simulink model "msd_sl_ctl"  (R2021b)
settings: Solver=VariableStepAuto  StartTime=0.0  StopTime=20.0  RelTol=1e-3
values from neighbouring files (symbols this model uses):
  A = [0 1; -k/m -c/m]    [msd_sl_ctrl_design.m]
  B = [0; 1/m]    [msd_sl_ctrl_design.m]
  K1 = 5    [msd_sl_ctrl_design.m]
  S = smcplace(A,B,P)    [msd_sl_ctrl_design.m]    (also in smcplace.m = [place(A11,A12,P) eye(Bcol)])
settings Model: Creator=shohei  LastModifiedBy=shohei

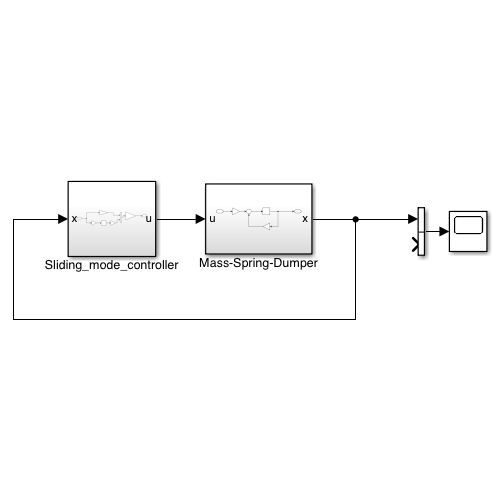
[thumbnail: Simulink's stored preview of the top-level diagram]
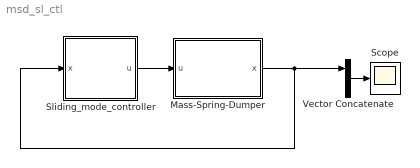
== system msd_sl_ctl ==
  Mass-Spring-Dumper : Subsystem
  Scope : Scope
  Sliding_mode_controller : Subsystem
  Vector Concatenate : Concatenate
  wires:
  Mass-Spring-Dumper/1(x) -> Sliding_mode_controller/1(x), Vector Concatenate/1
  Sliding_mode_controller/1(u) -> Mass-Spring-Dumper/1(u)
  Vector Concatenate/1 -> Scope/1

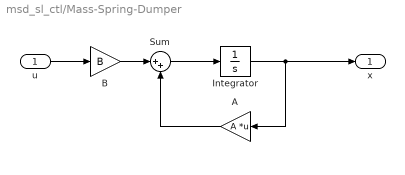
== system msd_sl_ctl/Mass-Spring-Dumper ==
  u : Inport
  A : Gain  Gain=A  Multiplication=Matrix(K*u)
  B : Gain  Gain=B
  Integrator : Integrator
  Sum : Sum  Inputs=|++
  x : Outport
  wires:
  u/1 -> B/1
  Sum/1 -> Integrator/1
  A/1 -> Sum/2
  Integrator/1 -> x/1, A/1
  B/1 -> Sum/1

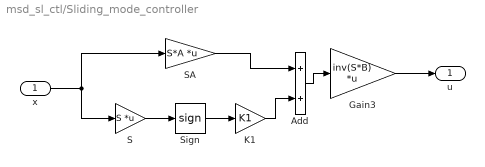
== system msd_sl_ctl/Sliding_mode_controller ==
  x : Inport
  Add : Sum
  Gain3 : Gain  Gain=inv(S*B)  Multiplication=Matrix(K*u)
  K1 : Gain  Gain=K1
  S : Gain  Gain=S  Multiplication=Matrix(K*u)
  SA : Gain  Gain=S*A  Multiplication=Matrix(K*u)
  Sign : Signum
  u : Outport
  wires:
  Add/1 -> Gain3/1
  x/1 -> SA/1, S/1
  K1/1 -> Add/2
  S/1 -> Sign/1
  Gain3/1 -> u/1
  Sign/1 -> K1/1
  SA/1 -> Add/1
